simulink model "lab2_malha_aberta"  (R2025a)
settings: Solver=ode4  StartTime=0.0  StopTime=10.0  FixedStep=0.01  RelTol=1e-3
values from neighbouring files (symbols this model uses):
  d1_final_value = 0    [matlab_script.m]
  d1_initial_value = 0    [matlab_script.m]
  d1_step_time = 0    [matlab_script.m]
  d2_final_value = 0    [matlab_script.m]
  d2_initial_value = 0    [matlab_script.m]
  d2_step_time = 0    [matlab_script.m]
  final_value = 1    [matlab_script.m]
  initial_value = 0    [matlab_script.m]
  step_time = 1    [matlab_script.m]
libraries: cstblocks x4
settings Model: Creator=breno

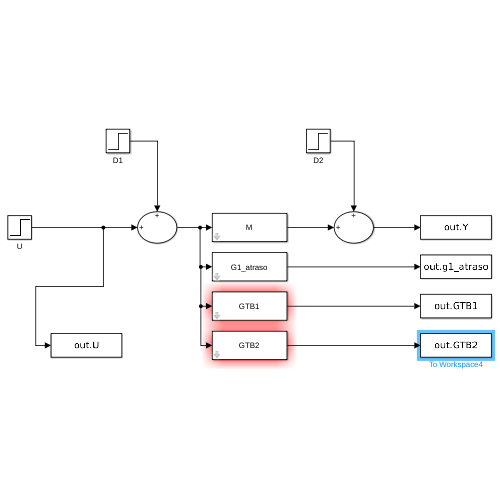
[thumbnail: Simulink's stored preview of the top-level diagram]
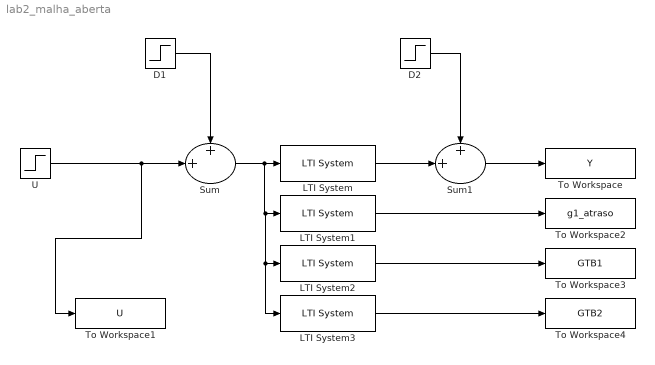
== system lab2_malha_aberta ==
  D1 : Step  Time=d1_step_time  Before=d1_initial_value  After=d1_final_value  SampleTime=0
  D2 : Step  Time=d2_step_time  Before=d2_initial_value  After=d2_final_value  SampleTime=0
  LTI System : cstblocks/LTI System  sys=M  IC=[]  PadeOrder=0
  LTI System1 : cstblocks/LTI System  sys=G1_atraso  IC=[]  PadeOrder=0
  LTI System2 : cstblocks/LTI System  sys=GTB1  IC=[]  PadeOrder=0
  LTI System3 : cstblocks/LTI System  sys=GTB2  IC=[]  PadeOrder=0
  Sum : Sum  Inputs=++|
  Sum1 : Sum  Inputs=++|
  To Workspace : ToWorkspace  VariableName=Y  SaveFormat=Timeseries  SampleTime=-1
  To Workspace1 : ToWorkspace  VariableName=U  SaveFormat=Timeseries  SampleTime=-1
  To Workspace2 : ToWorkspace  VariableName=g1_atraso  SaveFormat=Timeseries  SampleTime=-1
  To Workspace3 : ToWorkspace  VariableName=GTB1  SaveFormat=Timeseries  SampleTime=-1
  To Workspace4 : ToWorkspace  VariableName=GTB2  SaveFormat=Timeseries  SampleTime=-1
  U : Step  Time=step_time  Before=initial_value  After=final_value  SampleTime=0
  wires:
  Sum/1 -> LTI System3/1, LTI System2/1, LTI System1/1, LTI System/1
  LTI System/1 -> Sum1/2
  D1/1 -> Sum/1
  U/1 -> Sum/2, To Workspace1/1
  D2/1 -> Sum1/1
  Sum1/1 -> To Workspace/1
  LTI System1/1 -> To Workspace2/1
  LTI System2/1 -> To Workspace3/1
  LTI System3/1 -> To Workspace4/1
